simulink model "ModelPreAmp2"  (R2022b)
settings: Solver=FixedStepDiscrete  StartTime=0.0  StopTime=1  RelTol=1e-3  EnableMultiTasking=on
InitFcn:
  | % Initialize model
  | run(['ModelInit.m']);
  | 
  | % load library data
  | GainLibrary_data;
StartFcn:
  | % make sure all the simulated RTC requests are found
  | %RTC_SIM_OBJ.ValidateREQs();
model workspace (MAT data in the model file):
  PreampVolumeTable_Idx : Simulink.Signal (value not decoded)
  Range : Simulink.Signal (value not decoded)
  Table_Idx : Simulink.Signal (value not decoded)
undefined symbols (not defined in the file): MedusaConfig, MuteRamper, MuteRamperBtc, numAudioIn, sys_defs
libraries: FeaturePath x12, RTC x5, dspindex x5, SampleRateConverter x4, EdgePorts x2, FadeRamper x2, AudioStats x2, HandyTextFile x2, SleepingBeauty x2, dspsrcs4 x2, Router x1, FadeControl x1
(part 2 of 2)

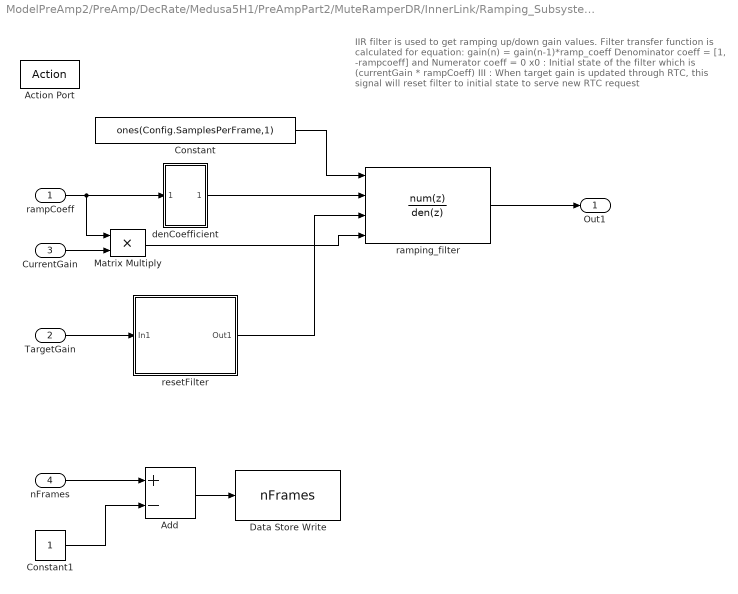
== system ModelPreAmp2/PreAmp/DecRate/Medusa5H1/PreAmpPart2/MuteRamperDR/InnerLink/Ramping_Subsystem/RampingGain/ifActionSubsystem ==
  note: IIR filter is used to get ramping up/down gain values. Filter transfer function
      |  is calculated for equation:
      | 	gain(n) = gain(n-1)*ramp_coeff
      |
      | Denominator coeff  = [1, -rampcoeff]  and Numerator coeff = 0
      | x0 : Initial state of the filter which is (currentGain * rampCoeff)
      | III : When target gain is updated through RTC, this signal will reset filter to
      | 	initial state to serve new RTC request
  rampCoeff : Inport
  TargetGain : Inport  Port=2
  CurrentGain : Inport  Port=3
  nFrames : Inport  Port=4
  Action Port : ActionPort  ActionPortLabel=if((u1>u2) & (u3>0))
  Add : Sum  Inputs=+-
  Constant : Constant  Value=ones(Config.SamplesPerFrame,1)  VectorParams1D=off  OutDataTypeStr=single
  Constant1 : Constant  OutDataTypeStr=single
  Data Store Write : DataStoreWrite  DataStoreName=nFrames  IndexOptions=Index vector (dialog)  Indices=1  OutputSizes=1
  Matrix Multiply : Product
  denCoefficient : Subsystem
  ramping_filter : DiscreteFilter  Numerator=0  DenominatorSource=Input port  Denominator=[1 -1.0003]  InitialStatesSource=Input port  InitialStates=1.0003  InputProcessing=Columns as channels (frame based)  ExternalReset=Level hold  FilterStructure=Direct form II transposed  a0EqualsOne=on
      settings: InputPortMap=u0,p3,r7,p5
  resetFilter : Subsystem
  Out1 : Outport
  wires:
  nFrames/1 -> Add/1
  Constant1/1 -> Add/2
  Add/1 -> Data Store Write/1
  Matrix Multiply/1 -> ramping_filter/4
  CurrentGain/1 -> Matrix Multiply/2
  ramping_filter/1 -> Out1/1
  Constant/1 -> ramping_filter/1
  rampCoeff/1 -> Matrix Multiply/1, denCoefficient/1(In1)
  resetFilter/1(Out1) -> ramping_filter/3
  denCoefficient/1(Out1) -> ramping_filter/2
  TargetGain/1 -> resetFilter/1(In1)

== system ModelPreAmp2/PreAmp/DecRate/Medusa5H1/PreAmpPart2/MuteRamperDR/InnerLink/Ramping_Subsystem/applyGain/For Each Subsystem ==
  In1 : Inport  Partition=on  PartitionDimension=1  PartitionWidth=1  PartitionOffset=0
  In2 : Inport  Port=2  Partition=on  PartitionDimension=1  PartitionWidth=1  PartitionOffset=0
  For Each : ForEach  DisableCoverage=on
  Multiply : Product  Multiplication=Matrix(*)
  Out1 : Outport  ConcatenationDimension=1
  wires:
  Multiply/1 -> Out1/1
  In2/1 -> Multiply/2
  In1/1 -> Multiply/1

== system ModelPreAmp2/PreAmp/DecRate/Medusa5H1/PreAmpPart2/MuteRamperFR/InnerLink/Ramping_Subsystem/RampingGain/elseActionSubsystem ==
  In1 : Inport
  Action Port : ActionPort  ActionPortLabel=else
  Constant : Constant  Value=ones(Config.SamplesPerFrame,1)  VectorParams1D=off  OutDataTypeStr=single
  Multiply : Product
  Out1 : Outport  VectorParamsAs1DForOutWhenUnconnected=off
  wires:
  Constant/1 -> Multiply/1
  In1/1 -> Multiply/2
  Multiply/1 -> Out1/1

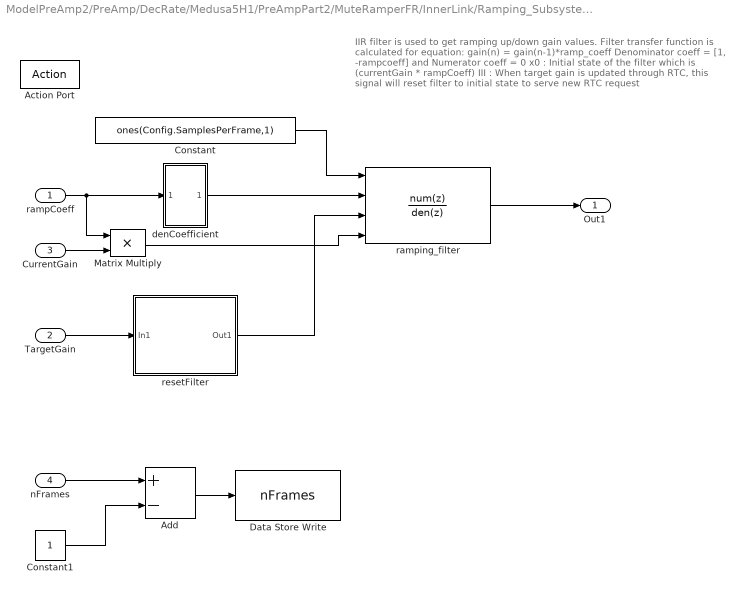
== system ModelPreAmp2/PreAmp/DecRate/Medusa5H1/PreAmpPart2/MuteRamperFR/InnerLink/Ramping_Subsystem/RampingGain/ifActionSubsystem ==
  note: IIR filter is used to get ramping up/down gain values. Filter transfer function
      |  is calculated for equation:
      | 	gain(n) = gain(n-1)*ramp_coeff
      |
      | Denominator coeff  = [1, -rampcoeff]  and Numerator coeff = 0
      | x0 : Initial state of the filter which is (currentGain * rampCoeff)
      | III : When target gain is updated through RTC, this signal will reset filter to
      | 	initial state to serve new RTC request
  rampCoeff : Inport
  TargetGain : Inport  Port=2
  CurrentGain : Inport  Port=3
  nFrames : Inport  Port=4
  Action Port : ActionPort  ActionPortLabel=if((u1>u2) & (u3>0))
  Add : Sum  Inputs=+-
  Constant : Constant  Value=ones(Config.SamplesPerFrame,1)  VectorParams1D=off  OutDataTypeStr=single
  Constant1 : Constant  OutDataTypeStr=single
  Data Store Write : DataStoreWrite  DataStoreName=nFrames  IndexOptions=Index vector (dialog)  Indices=1  OutputSizes=1
  Matrix Multiply : Product
  denCoefficient : Subsystem
  ramping_filter : DiscreteFilter  Numerator=0  DenominatorSource=Input port  Denominator=[1 -1.0003]  InitialStatesSource=Input port  InitialStates=1.0003  InputProcessing=Columns as channels (frame based)  ExternalReset=Level hold  FilterStructure=Direct form II transposed  a0EqualsOne=on
      settings: InputPortMap=u0,p3,r7,p5
  resetFilter : Subsystem
  Out1 : Outport
  wires:
  nFrames/1 -> Add/1
  Constant1/1 -> Add/2
  Add/1 -> Data Store Write/1
  Matrix Multiply/1 -> ramping_filter/4
  CurrentGain/1 -> Matrix Multiply/2
  ramping_filter/1 -> Out1/1
  Constant/1 -> ramping_filter/1
  rampCoeff/1 -> Matrix Multiply/1, denCoefficient/1(In1)
  resetFilter/1(Out1) -> ramping_filter/3
  denCoefficient/1(Out1) -> ramping_filter/2
  TargetGain/1 -> resetFilter/1(In1)

== system ModelPreAmp2/PreAmp/DecRate/Medusa5H1/PreAmpPart2/MuteRamperFR/InnerLink/Ramping_Subsystem/applyGain/For Each Subsystem ==
  In1 : Inport  Partition=on  PartitionDimension=1  PartitionWidth=1  PartitionOffset=0
  In2 : Inport  Port=2  Partition=on  PartitionDimension=1  PartitionWidth=1  PartitionOffset=0
  For Each : ForEach  DisableCoverage=on
  Multiply : Product  Multiplication=Matrix(*)
  Out1 : Outport  ConcatenationDimension=1
  wires:
  Multiply/1 -> Out1/1
  In2/1 -> Multiply/2
  In1/1 -> Multiply/1

== system ModelPreAmp2/PreAmp/DecRate/Medusa5H1/PreAmpPart2/MuteRamperDR/InnerLink/Ramping_Subsystem/RampingGain/ifActionSubsystem/denCoefficient ==
  In1 : Inport
  Constant : Constant  Value=-1  OutDataTypeStr=single
  Constant3 : Constant  OutDataTypeStr=single
  Matrix Concatenate : Concatenate  Mode=Multidimensional array  ConcatenateDimension=2
  Multiply : Product
  Out1 : Outport  VectorParamsAs1DForOutWhenUnconnected=off
  wires:
  In1/1 -> Multiply/2
  Multiply/1 -> Matrix Concatenate/2
  Constant/1 -> Multiply/1
  Matrix Concatenate/1 -> Out1/1
  Constant3/1 -> Matrix Concatenate/1

== system ModelPreAmp2/PreAmp/DecRate/Medusa5H1/PreAmpPart2/MuteRamperDR/InnerLink/Ramping_Subsystem/RampingGain/ifActionSubsystem/resetFilter ==
  In1 : Inport
  Add2 : Sum  Inputs=+-
  Delay : Delay  DelayLength=1
  If : If  IfExpression=u1 == 0
  If Action Subsystem : Subsystem  TreatAsAtomicUnit=on
  If Action Subsystem1 : Subsystem  TreatAsAtomicUnit=on
  Merge : Merge
  Out1 : Outport  VectorParamsAs1DForOutWhenUnconnected=off
  wires:
  Merge/1 -> Out1/1
  If Action Subsystem1/1(Out1) -> Merge/2
  If Action Subsystem/1(Out1) -> Merge/1
  If/2 -> If Action Subsystem1/Action
  If/1 -> If Action Subsystem/Action
  In1/1 -> Delay/1, Add2/1
  Delay/1 -> Add2/2
  Add2/1 -> If/1

== system ModelPreAmp2/PreAmp/DecRate/Medusa5H1/PreAmpPart2/MuteRamperFR/InnerLink/Ramping_Subsystem/RampingGain/ifActionSubsystem/denCoefficient ==
  In1 : Inport
  Constant : Constant  Value=-1  OutDataTypeStr=single
  Constant3 : Constant  OutDataTypeStr=single
  Matrix Concatenate : Concatenate  Mode=Multidimensional array  ConcatenateDimension=2
  Multiply : Product
  Out1 : Outport  VectorParamsAs1DForOutWhenUnconnected=off
  wires:
  In1/1 -> Multiply/2
  Multiply/1 -> Matrix Concatenate/2
  Constant/1 -> Multiply/1
  Matrix Concatenate/1 -> Out1/1
  Constant3/1 -> Matrix Concatenate/1

== system ModelPreAmp2/PreAmp/DecRate/Medusa5H1/PreAmpPart2/MuteRamperFR/InnerLink/Ramping_Subsystem/RampingGain/ifActionSubsystem/resetFilter ==
  In1 : Inport
  Add2 : Sum  Inputs=+-
  Delay : Delay  DelayLength=1
  If : If  IfExpression=u1 == 0
  If Action Subsystem : Subsystem  TreatAsAtomicUnit=on
  If Action Subsystem1 : Subsystem  TreatAsAtomicUnit=on
  Merge : Merge
  Out1 : Outport  VectorParamsAs1DForOutWhenUnconnected=off
  wires:
  Merge/1 -> Out1/1
  If Action Subsystem1/1(Out1) -> Merge/2
  If Action Subsystem/1(Out1) -> Merge/1
  If/2 -> If Action Subsystem1/Action
  If/1 -> If Action Subsystem/Action
  In1/1 -> Delay/1, Add2/1
  Delay/1 -> Add2/2
  Add2/1 -> If/1

== system ModelPreAmp2/PreAmp/DecRate/Medusa5H1/PreAmpPart2/MuteRamperDR/InnerLink/Ramping_Subsystem/RampingGain/ifActionSubsystem/resetFilter/If Action Subsystem ==
  Action Port : ActionPort  ActionPortLabel=if(u1 == 0)
  Constant : Constant  Value=0  OutDataTypeStr=boolean
  Out1 : Outport  VectorParamsAs1DForOutWhenUnconnected=off
  wires:
  Constant/1 -> Out1/1

== system ModelPreAmp2/PreAmp/DecRate/Medusa5H1/PreAmpPart2/MuteRamperDR/InnerLink/Ramping_Subsystem/RampingGain/ifActionSubsystem/resetFilter/If Action Subsystem1 ==
  Action Port : ActionPort  ActionPortLabel=else
  Constant : Constant  OutDataTypeStr=boolean
  Out1 : Outport  VectorParamsAs1DForOutWhenUnconnected=off
  wires:
  Constant/1 -> Out1/1

== system ModelPreAmp2/PreAmp/DecRate/Medusa5H1/PreAmpPart2/MuteRamperFR/InnerLink/Ramping_Subsystem/RampingGain/ifActionSubsystem/resetFilter/If Action Subsystem ==
  Action Port : ActionPort  ActionPortLabel=if(u1 == 0)
  Constant : Constant  Value=0  OutDataTypeStr=boolean
  Out1 : Outport  VectorParamsAs1DForOutWhenUnconnected=off
  wires:
  Constant/1 -> Out1/1

== system ModelPreAmp2/PreAmp/DecRate/Medusa5H1/PreAmpPart2/MuteRamperFR/InnerLink/Ramping_Subsystem/RampingGain/ifActionSubsystem/resetFilter/If Action Subsystem1 ==
  Action Port : ActionPort  ActionPortLabel=else
  Constant : Constant  OutDataTypeStr=boolean
  Out1 : Outport  VectorParamsAs1DForOutWhenUnconnected=off
  wires:
  Constant/1 -> Out1/1

== matlab function ModelPreAmp2/NEAR/MATLAB Function ==
  data: u input; y output
function y = fcn(u)

y = u;

== matlab function ModelPreAmp2/PreAmp/Reset/MATLAB Function ==
  events: trigger input FUNCTION_CALL_EVENT
function fcn()

if coder.target('Rtw')
    coder.ceval('Model_Target_DRFDP_initialize');
    coder.ceval('Model_Target_FRFDP_initialize');
    coder.ceval('Model_Target_ExpandTailComponents_initialize');
    coder.ceval('Model_Target_TrebleandSurroundDelays_initialize');
    coder.ceval('Model_Target_Medusa5H1Part3_initialize');
    coder.ceval('Model_Target_Subsystem_initialize');
    
    coder.ceval('Model_Target_PreAmpPart1_Start');
    coder.ceval('Model_Target_SRCIn_Start');
%     coder.ceval('Model_Target_AudioPilot35_Start');
    coder.ceval('Model_Target_Medusa5H1Part1_Start');
    coder.ceval('Model_Target_Medusa5H1Part2_Start');
    coder.ceval('Model_Target_Medusa5H1Part3_Start');

    coder.ceval('Model_Target_PreAmpPart1_Init');
    coder.ceval('Model_Target_PreAmpPart2_Init');
%     coder.ceval('Model_Target_SRCIn_Init');
%     coder.ceval('Model_Target_SRCOut_Init');
%     coder.ceval('Model_Target_AudioPilot35_Init');
    coder.ceval('Model_Target_Medusa5H1Part1_Init');
    coder.ceval('Model_Target_Medusa5H1Part2_Init');
    coder.ceval('Model_Target_Medusa5H1Part3_Init');
end

== matlab function ModelPreAmp2/InputSelect/Reset/MATLAB Function ==
  events: trigger input FUNCTION_CALL_EVENT
function fcn()

if coder.target('Rtw')
    coder.ceval('Model_Target_InputSelect_Init');
end

== matlab function ModelPreAmp2/PreAmp/DecRate/Medusa5H1/PreAmpPart2/MATLAB Function ==
  events: trigger input FUNCTION_CALL_EVENT
function fcn()

if coder.target('Rtw')
  
end

== matlab function ModelPreAmp2/PostProcess/Reset/MATLAB Function ==
  events: trigger input FUNCTION_CALL_EVENT
function fcn()

if coder.target('Rtw')
    coder.ceval('Model_Target_PostProcess_initialize');
    coder.ceval('Model_Target_PostProcess_Start');
    coder.ceval('Model_Target_PostProcess_Init');
end

== matlab function ModelPreAmp2/PreAmp/DecRate/Medusa5H1/PreAmpPart2/MuteRamperDR/InnerLink/TriggeredFunction ==
  data: done output; targetLinearGain data_store_memory; currentGain data_store_memory
  events: trigger input FUNCTION_CALL_EVENT
function done = NotificationCheck()
% Function to check whether the ramp has completed. 
% If so, send out TRUE

global targetLinearGain;
global currentGain;

% Assume the work is complete until proven otherwise
done = true;
if (targetLinearGain ~= currentGain)
   done = false; % just proved otherwise
end

== matlab function ModelPreAmp2/PreAmp/DecRate/Medusa5H1/PreAmpPart2/MuteRamperDR/InnerLink/get_ramp_coeffs ==
  data: currentGainValue input; muteSwitch input; ramping_coeff output; rampingRate_dBPerSec input; rampingTime_ms input; Fs_Hz input; silentGainLinear parameter; targetLinearGain data_store_memory; nFrames data_store_memory; frameSize parameter
  events: trigger input FUNCTION_CALL_EVENT
function ramping_coeff = fcn(currentGainValue, muteSwitch, rampingRate_dBPerSec,rampingTime_ms, Fs_Hz, silentGainLinear, frameSize)

global targetLinearGain
global nFrames
targetLinearGain = single(1.0);

if muteSwitch
    targetLinearGain = single(max(0, silentGainLinear));
end

% % Nudge the gain values a bit if they are sitting at zero.
% % If current gain is zero, replace with a value very close to zero. What we
% % really want is a value which is on the edge of perception - not too small
% % or large. If the value is too small, we'll waste some of our ramp time
% % in perceived silence. If the value is too large, the audio will lurch
% % into perceptability at the start of the ramp.
% % So, 'max(currentGainValue, silentGainLinear)' & 'max(TargetGain, silentGainLinear)' are
% % used in equations

% In order to have the desired ramp time, the slope must vary dependent
% on the gain difference between target and current value.
% Equivalent ramp rate is therefore calculated as follows:

if (rampingRate_dBPerSec)
    currentGain_db = 20*log10(max(currentGainValue, silentGainLinear));
    targetGain_db = 20*log10( targetLinearGain);
    diff = abs(currentGain_db - targetGain_db);
    rampingTime_ms = diff / single(rampingRate_dBPerSec) * 1000;
end

quantum_ms = 1000 * frameSize / Fs_Hz;
numFrames = rampingTime_ms / quantum_ms;
% Do a ceil rather than a round to insure that we create enough
% frames. i.e. a fraction of a frame is promoted to an addition frame
nFrames = max (1, ceil(numFrames));
quantized_rampTime_ms = nFrames * quantum_ms;
   
% In order to have the desired ramp time, the slope must vary dependent
% on the gain differencebetween target and current value.
% Ramper's coefficient is therefore calculated as follows:
%
%   TargetGain = CurrentGain *( RampCoef ^ (Fs*RampTime_ms/1000) )
%
% therefore...
%
%                     log(TargetGain/CurrentGain)
%   log(RampCoef) = ------------------------------
%                        Fs*(RampTime_ms/1000)
%
ramping_coeff= exp(log( targetLinearGain /max(currentGainValue, silentGainLinear) ) / (Fs_Hz * quantized_rampTime_ms / 1000));

== matlab function ModelPreAmp2/PreAmp/DecRate/Medusa5H1/PreAmpPart2/MuteRamperFR/InnerLink/TriggeredFunction ==
  data: done output; targetLinearGain data_store_memory; currentGain data_store_memory
  events: trigger input FUNCTION_CALL_EVENT
function done = NotificationCheck()
% Function to check whether the ramp has completed. 
% If so, send out TRUE

global targetLinearGain;
global currentGain;

% Assume the work is complete until proven otherwise
done = true;
if (targetLinearGain ~= currentGain)
   done = false; % just proved otherwise
end

== matlab function ModelPreAmp2/PreAmp/DecRate/Medusa5H1/PreAmpPart2/MuteRamperFR/InnerLink/get_ramp_coeffs ==
  data: currentGainValue input; muteSwitch input; ramping_coeff output; rampingRate_dBPerSec input; rampingTime_ms input; Fs_Hz input; silentGainLinear parameter; targetLinearGain data_store_memory; nFrames data_store_memory; frameSize parameter
  events: trigger input FUNCTION_CALL_EVENT
function ramping_coeff = fcn(currentGainValue, muteSwitch, rampingRate_dBPerSec,rampingTime_ms, Fs_Hz, silentGainLinear, frameSize)

global targetLinearGain
global nFrames
targetLinearGain = single(1.0);

if muteSwitch
    targetLinearGain = single(max(0, silentGainLinear));
end

% % Nudge the gain values a bit if they are sitting at zero.
% % If current gain is zero, replace with a value very close to zero. What we
% % really want is a value which is on the edge of perception - not too small
% % or large. If the value is too small, we'll waste some of our ramp time
% % in perceived silence. If the value is too large, the audio will lurch
% % into perceptability at the start of the ramp.
% % So, 'max(currentGainValue, silentGainLinear)' & 'max(TargetGain, silentGainLinear)' are
% % used in equations

% In order to have the desired ramp time, the slope must vary dependent
% on the gain difference between target and current value.
% Equivalent ramp rate is therefore calculated as follows:

if (rampingRate_dBPerSec)
    currentGain_db = 20*log10(max(currentGainValue, silentGainLinear));
    targetGain_db = 20*log10( targetLinearGain);
    diff = abs(currentGain_db - targetGain_db);
    rampingTime_ms = diff / single(rampingRate_dBPerSec) * 1000;
end

quantum_ms = 1000 * frameSize / Fs_Hz;
numFrames = rampingTime_ms / quantum_ms;
% Do a ceil rather than a round to insure that we create enough
% frames. i.e. a fraction of a frame is promoted to an addition frame
nFrames = max (1, ceil(numFrames));
quantized_rampTime_ms = nFrames * quantum_ms;
   
% In order to have the desired ramp time, the slope must vary dependent
% on the gain differencebetween target and current value.
% Ramper's coefficient is therefore calculated as follows:
%
%   TargetGain = CurrentGain *( RampCoef ^ (Fs*RampTime_ms/1000) )
%
% therefore...
%
%                     log(TargetGain/CurrentGain)
%   log(RampCoef) = ------------------------------
%                        Fs*(RampTime_ms/1000)
%
ramping_coeff= exp(log( targetLinearGain /max(currentGainValue, silentGainLinear) ) / (Fs_Hz * quantized_rampTime_ms / 1000));
